simulink model "condensertest"  (R2018b)
settings: Solver=VariableStepAuto  StartTime=0.0  StopTime=10.0  RelTol=1e-3
settings Model: Creator=sofi  LastModifiedBy=art58

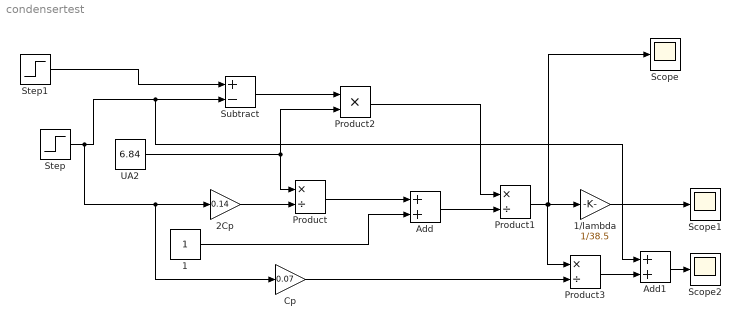
== system condensertest ==
  1 : Constant
  1/lambda : Gain  Gain=1/38.5
  2Cp : Gain  Gain=0.14
  Add : Sum
  Add1 : Sum
  Cp : Gain  Gain=0.07
  Product : Product  Inputs=*/
  Product1 : Product  Inputs=*/
  Product2 : Product
  Product3 : Product  Inputs=*/
  Scope : Scope
  Scope1 : Scope
  Scope2 : Scope
  Step : Step  Before=0.1  After=2  SampleTime=0
  Step1 : Step  Before=0.1  SampleTime=0
  Subtract : Sum  Inputs=+-
  UA2 : Constant  Value=6.84
  wires:
  2Cp/1 -> Product/2
  UA2/1 -> Product/1, Product2/2
  Product/1 -> Add/1
  1/1 -> Add/2
  Add/1 -> Product1/2
  Subtract/1 -> Product2/1
  Product2/1 -> Product1/1
  Product1/1 -> Scope/1, 1/lambda/1, Product3/1
  1/lambda/1 -> Scope1/1
  Step/1 -> Cp/1, 2Cp/1, Add1/1, Subtract/2
  Cp/1 -> Product3/2
  Product3/1 -> Add1/2
  Add1/1 -> Scope2/1
  Step1/1 -> Subtract/1
